simulink model "DOF4_model"  (R2022b)
settings: Solver=FixedStepAuto  StartTime=0.0  StopTime=100  FixedStep=0.005  RelTol=1e-3
values from neighbouring files (symbols this model uses):
  a = 1.80    (= 1.8)    [DOF4_model_parameters.m]
undefined symbols (not defined in the file or in its folder): b, cfdamper, crdamper, F0f, F0r, g, I, kfspring, krspring, ktyre, ms, musf, musr, z0ftyre, z0rtyre
libraries: simulink x1
settings Model: Creator=webstert  LastModifiedBy=webstert

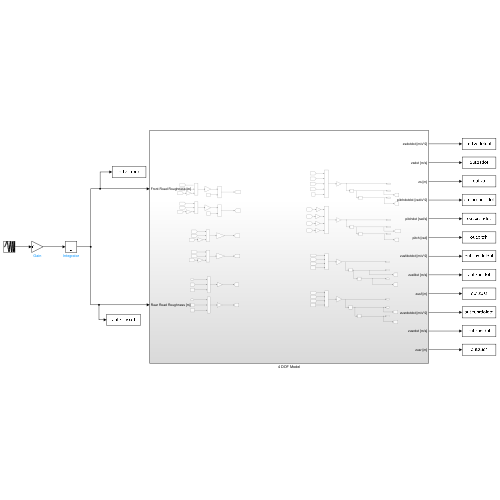
[thumbnail: Simulink's stored preview of the top-level diagram]
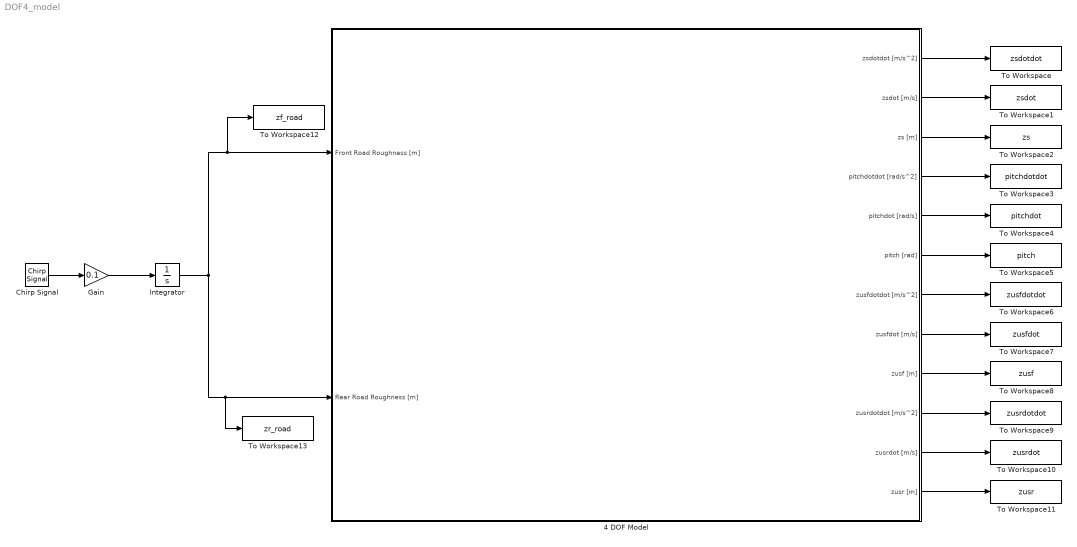
== system DOF4_model ==
  4 DOF Model : Subsystem
  Chirp Signal : simulink/Sources/Chirp Signal  f1=0.1  T=100  f2=50
  Gain : Gain  Gain=0.1
  Integrator : Integrator
  To Workspace : ToWorkspace  VariableName=zsdotdot  SaveFormat=Timeseries  SampleTime=-1
  To Workspace1 : ToWorkspace  VariableName=zsdot  SaveFormat=Timeseries  SampleTime=-1
  To Workspace10 : ToWorkspace  VariableName=zusrdot  SaveFormat=Timeseries  SampleTime=-1
  To Workspace11 : ToWorkspace  VariableName=zusr  SaveFormat=Timeseries  SampleTime=-1
  To Workspace12 : ToWorkspace  VariableName=zf_road  SaveFormat=Timeseries  SampleTime=-1
  To Workspace13 : ToWorkspace  VariableName=zr_road  SaveFormat=Timeseries  SampleTime=-1
  To Workspace2 : ToWorkspace  VariableName=zs  SaveFormat=Timeseries  SampleTime=-1
  To Workspace3 : ToWorkspace  VariableName=pitchdotdot  SaveFormat=Timeseries  SampleTime=-1
  To Workspace4 : ToWorkspace  VariableName=pitchdot  SaveFormat=Timeseries  SampleTime=-1
  To Workspace5 : ToWorkspace  VariableName=pitch  SaveFormat=Timeseries  SampleTime=-1
  To Workspace6 : ToWorkspace  VariableName=zusfdotdot  SaveFormat=Timeseries  SampleTime=-1
  To Workspace7 : ToWorkspace  VariableName=zusfdot  SaveFormat=Timeseries  SampleTime=-1
  To Workspace8 : ToWorkspace  VariableName=zusf  SaveFormat=Timeseries  SampleTime=-1
  To Workspace9 : ToWorkspace  VariableName=zusrdotdot  SaveFormat=Timeseries  SampleTime=-1
  wires:
  4 DOF Model/1(zsdotdot [m/s^2]) -> To Workspace/1
  4 DOF Model/2(zsdot [m/s]) -> To Workspace1/1
  4 DOF Model/3(zs [m]) -> To Workspace2/1
  4 DOF Model/4(pitchdotdot [rad/s^2]) -> To Workspace3/1
  4 DOF Model/5(pitchdot [rad/s]) -> To Workspace4/1
  4 DOF Model/6(pitch [rad]) -> To Workspace5/1
  4 DOF Model/7(zusfdotdot [m/s^2]) -> To Workspace6/1
  4 DOF Model/8(zusfdot [m/s]) -> To Workspace7/1
  4 DOF Model/9(zusf [m]) -> To Workspace8/1
  4 DOF Model/10(zusrdotdot [m/s^2]) -> To Workspace9/1
  4 DOF Model/11(zusrdot [m/s]) -> To Workspace10/1
  4 DOF Model/12(zusr [m]) -> To Workspace11/1
  Chirp Signal/1 -> Gain/1
  Gain/1 -> Integrator/1
  Integrator/1 -> To Workspace12/1, 4 DOF Model/1(Front Road Roughness [m]), To Workspace13/1, 4 DOF Model/2(Rear Road Roughness [m])

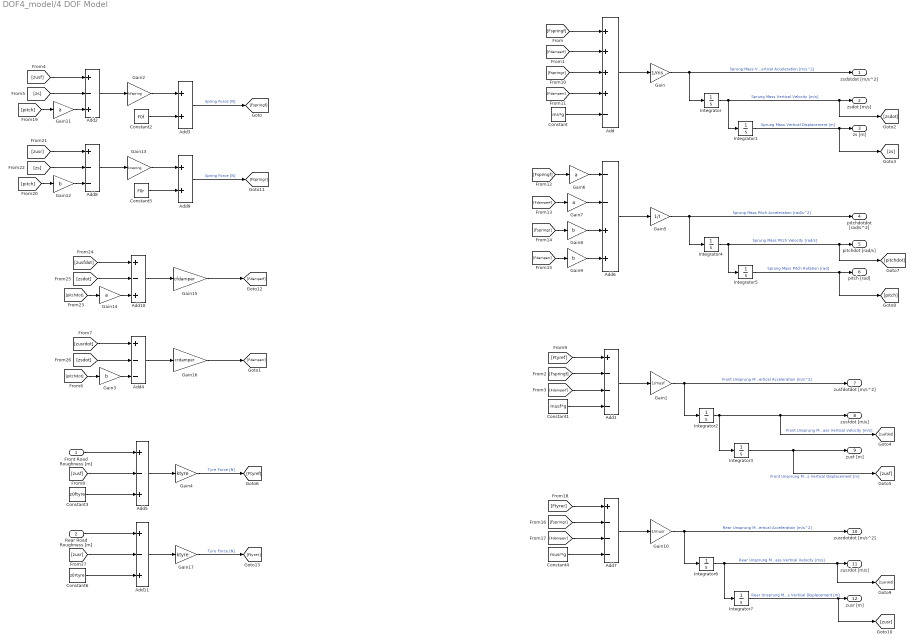
== system DOF4_model/4 DOF Model ==
  Front Road Roughness [m] : Inport
  Rear Road Roughness [m] : Inport  Port=2
  Add : Sum  Inputs=++++-
  Add1 : Sum  Inputs=+---
  Add{2,5,10..11} (4 alike) : Sum  Inputs=+-+
  Add3 : Sum
  Add4 : Sum  Inputs=+--
  Add6 : Sum  Inputs=--++
  Add7 : Sum  Inputs=+---
  Add8 : Sum  Inputs=+--
  Add9 : Sum
  Constant : Constant  Value=ms*g
  Constant1 : Constant  Value=musf*g
  Constant2 : Constant  Value=F0f
  Constant3 : Constant  Value=z0ftyre
  Constant4 : Constant  Value=musr*g
  Constant5 : Constant  Value=F0r
  Constant6 : Constant  Value=z0rtyre
  Gain : Gain  Gain=1/ms
  Gain1 : Gain  Gain=1/musf
  Gain10 : Gain  Gain=1/musr
  Gain{6..7,11,14} (4 alike) : Gain  Gain=a
  Gain{3,8..9,12} (4 alike) : Gain  Gain=b
  Gain13 : Gain  Gain=krspring
  Gain15 : Gain  Gain=cfdamper
  Gain16 : Gain  Gain=crdamper
  Gain17 : Gain  Gain=ktyre
  Gain2 : Gain  Gain=kfspring
  Gain4 : Gain  Gain=ktyre
  Gain5 : Gain  Gain=1/I
  Integrator{,1..7} (8 alike) : Integrator
  zsdotdot [m/s^2] : Outport
  zsdot [m/s] : Outport  Port=2
  zs [m] : Outport  Port=3
  pitchdotdot [rad/s^2] : Outport  Port=4
  pitchdot [rad/s] : Outport  Port=5
  pitch [rad] : Outport  Port=6
  zusfdotdot [m/s^2] : Outport  Port=7
  zusfdot [m/s] : Outport  Port=8
  zusf [m] : Outport  Port=9
  zusrdotdot [m/s^2] : Outport  Port=10
  zusrdot [m/s] : Outport  Port=11
  zusr [m] : Outport  Port=12
  wires:
  [Fdamperf] -> Add/2
  [Fspringf] -> Add/1
  Gain4/1 -> [Ftyref]  "Tyre Force [N]"
  Front Road Roughness [m]/1 -> Add5/1
  Constant3/1 -> Add5/3
  Add2/1 -> Gain2/1
  [zs] -> Add2/2
  Add5/1 -> Gain4/1
  Add1/1 -> Gain1/1
  Integrator3/1 -> [zusf], zusf [m]/1  "Front Unsprung Mass Vertical Displacement [m]"
  [Fdamperf] -> Add1/3
  Gain1/1 -> zusfdotdot [m/s^2]/1, Integrator2/1  "Front Unsprung Mass Vertical Acceleration [m/s^2]"
  Integrator1/1 -> [zs], zs [m]/1  "Sprung Mass Vertical Displacement [m]"
  Add3/1 -> [Fspringf]  "Spring Force [N]"
  [Ftyref] -> Add1/1
  [Fspringf] -> Add1/2
  Constant1/1 -> Add1/4
  [zusf] -> Add5/2
  Constant/1 -> Add/5
  Integrator/1 -> [zsdot], zsdot [m/s]/1, Integrator1/1  "Sprung Mass Vertical Velocity [m/s]"
  Gain2/1 -> Add3/1
  Constant2/1 -> Add3/2
  Add/1 -> Gain/1
  Gain/1 -> Integrator/1, zsdotdot [m/s^2]/1  "Sprung Mass Vertical Acceleration [m/s^2]"
  Integrator2/1 -> [zusfdot], zusfdot [m/s]/1, Integrator3/1  "Front Unsprung Mass Vertical Velocity [m/s]"
  [zusf] -> Add2/1
  [Fspringr] -> Add/3
  [Fdamperr] -> Add/4
  [Fdamperr] -> Gain9/1
  [Fspringr] -> Gain8/1
  Gain5/1 -> pitchdotdot [rad/s^2]/1, Integrator4/1  "Sprung Mass Pitch Acceleration [rad/s^2]"
  Add6/1 -> Gain5/1
  Integrator4/1 -> Integrator5/1, pitchdot [rad/s]/1, [pitchdot]  "Sprung Mass Pitch Velocity [rad/s]"
  Integrator5/1 -> pitch [rad]/1, [pitch]  "Sprung Mass Pitch Rotation [rad]"
  [Fspringf] -> Gain6/1
  [Fdamperf] -> Gain7/1
  Gain6/1 -> Add6/1
  Gain7/1 -> Add6/2
  Gain8/1 -> Add6/3
  Gain9/1 -> Add6/4
  Integrator6/1 -> Integrator7/1, zusrdot [m/s]/1, [zusrdot]  "Rear Unsprung Mass Vertical Velocity [m/s]"
  Constant4/1 -> Add7/4
  [Fspringr] -> Add7/2
  [Ftyrer] -> Add7/1
  Gain10/1 -> Integrator6/1, zusrdotdot [m/s^2]/1  "Rear Unsprung Mass Vertical Acceleration [m/s^2]"
  [Fdamperr] -> Add7/3
  Integrator7/1 -> zusr [m]/1, [zusr]  "Rear Unsprung Mass Vertical Displacement [m]"
  Add7/1 -> Gain10/1
  [pitch] -> Gain11/1
  Gain11/1 -> Add2/3
  [zusr] -> Add8/1
  Gain13/1 -> Add9/1
  [zs] -> Add8/2
  Add8/1 -> Gain13/1
  Add9/1 -> [Fspringr]  "Spring Force [N]"
  [pitch] -> Gain12/1
  Gain12/1 -> Add8/3
  Constant5/1 -> Add9/2
  Gain14/1 -> Add10/3
  [pitchdot] -> Gain14/1
  [zusfdot] -> Add10/1
  [zsdot] -> Add10/2
  Add10/1 -> Gain15/1
  Gain15/1 -> [Fdamperf]
  Gain16/1 -> [Fdamperr]
  Add4/1 -> Gain16/1
  [zsdot] -> Add4/2
  [zusrdot] -> Add4/1
  [pitchdot] -> Gain3/1
  Gain3/1 -> Add4/3
  Add11/1 -> Gain17/1
  Constant6/1 -> Add11/3
  [zusr] -> Add11/2
  Gain17/1 -> [Ftyrer]  "Tyre Force [N]"
  Rear Road Roughness [m]/1 -> Add11/1
